simulink model "CSTR_sim_old"  (R2017a)
settings: Solver=ode8  StartTime=0.0  StopTime=t_end  FixedStep=Ts  RelTol=1e-3
values from neighbouring files (symbols this model uses):
  A = eval(A)    [linearisation.m]    (also in real_inverse.m = D * real( V' * diag( exp( j * angle( diag( V * D *  V.' ) ) )
  B = eval(B)    [linearisation.m]
  C = eval(C)    [linearisation.m]
  Ca = 1e-6    (= 1e-06)    [initialisation.m]    (also in linearisation.m = m.Ca; parameters.mat)
  Cb = 1e-6    (= 1e-06)    [initialisation.m]    (also in linearisation.m = m.Cb; parameters.mat)
  Fa0 = double(eval(S.Fa))    [linearisation.m]    (also in set_point.mat = 0.00260416666667)
  Fb0 = double(eval(S.Fb))    [linearisation.m]    (also in set_point.mat = 0.00572916666667)
  kv = 0.01    [initialisation.m]    (also in linearisation.m = m.kv; parameters.mat)
  kw = 1e-14    [initialisation.m]    (also in linearisation.m = m.kw; parameters.mat)
  tFa_down = 65000    [Simulation_Control_Off.m]
  tFa_up = 35000    [Simulation_Control_Off.m]
  tFb_down = 125000    [Simulation_Control_Off.m]
  tFb_up = 95000    [Simulation_Control_Off.m]
  V = 30    [initialisation.m]    (also in linearisation.m = m.V; parameters.mat)
  xa0 = 3.1250e-07    (= 3.125e-07)    [initialisation.m]    (also in linearisation.m = m.xa0; parameters.mat; set_point.mat)
  y = simdata.Data(:, 2)    [Simulation_Control_Off.m]    (also in initialisation.m = 7; linearisation.m = -log10(sqrt((xb - xa)^2/4 + kw) - (xb - xa)/2); parameters.mat = 7)
settings Model: Creator=Ivona  LastModifiedBy=Ivona

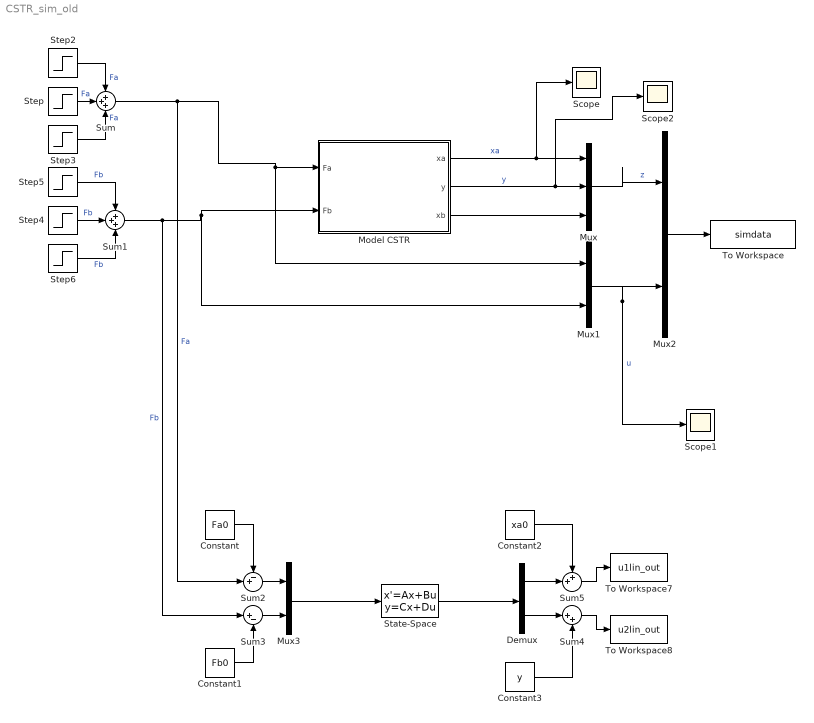
== system CSTR_sim_old ==
  Constant : Constant  Value=Fa0
  Constant1 : Constant  Value=Fb0
  Constant2 : Constant  Value=xa0
  Constant3 : Constant  Value=y
  Demux : Demux  Outputs=2
  Model CSTR : Subsystem
  Mux : Mux  Inputs=3
  Mux1 : Mux  Inputs=2
  Mux2 : Mux  Inputs=2
  Mux3 : Mux  Inputs=2
  Scope : Scope
  Scope1 : Scope
  Scope2 : Scope
  State-Space : StateSpace  A=A  B=B  C=C  D=[0 0;0 0]  X0=0
  Step : Step  Time=0  After=Fa0  SampleTime=0
  Step2 : Step  Time=tFa_up  After=0.1*Fa0  SampleTime=0
  Step3 : Step  Time=tFa_down  After=-0.1*Fa0  SampleTime=0
  Step4 : Step  Time=0  After=Fb0  SampleTime=0
  Step5 : Step  Time=tFb_up  After=0.1*Fb0  SampleTime=0
  Step6 : Step  Time=tFb_down  After=-0.1*Fb0  SampleTime=0
  Sum : Sum  Inputs=+++
  Sum1 : Sum  Inputs=+++
  Sum2 : Sum  Inputs=-+|
  Sum3 : Sum  Inputs=|+-
  Sum4 : Sum  Inputs=|++
  Sum5 : Sum  Inputs=++|
  To Workspace : ToWorkspace  VariableName=simdata  SaveFormat=Timeseries  SampleTime=-1
  To Workspace7 : ToWorkspace  VariableName=u1lin_out  SampleTime=-1
  To Workspace8 : ToWorkspace  VariableName=u2lin_out  SampleTime=-1
  wires:
  Model CSTR/1(xa) -> Mux/1, Scope/1  "xa"
  Model CSTR/2(y) -> Mux/2, Scope2/1  "y"
  Mux/1 -> Mux2/1  "z"
  Mux1/1 -> Scope1/1, Mux2/2  "u"
  Mux2/1 -> To Workspace/1
  Step/1 -> Sum/2  "Fa"
  Step2/1 -> Sum/1  "Fa"
  Step3/1 -> Sum/3  "Fa"
  Sum/1 -> Sum2/2, Mux1/1, Model CSTR/1(Fa)  "Fa"
  Step4/1 -> Sum1/2  "Fb"
  Step6/1 -> Sum1/3  "Fb"
  Step5/1 -> Sum1/1  "Fb"
  Sum1/1 -> Sum3/1, Mux1/2, Model CSTR/2(Fb)  "Fb"
  Model CSTR/3(xb) -> Mux/3
  Sum4/1 -> To Workspace8/1
  Constant2/1 -> Sum5/1
  Constant3/1 -> Sum4/2
  Constant1/1 -> Sum3/2
  Sum5/1 -> To Workspace7/1
  Constant/1 -> Sum2/1
  State-Space/1 -> Demux/1
  Demux/2 -> Sum4/1
  Sum2/1 -> Mux3/1
  Demux/1 -> Sum5/2
  Sum3/1 -> Mux3/2
  Mux3/1 -> State-Space/1

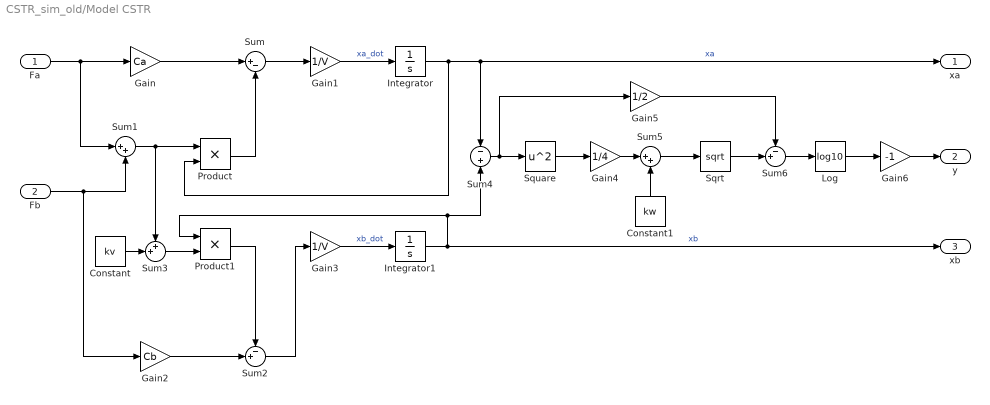
== system CSTR_sim_old/Model CSTR ==
  Fa : Inport
  Fb : Inport  Port=2
  Constant : Constant  Value=kv
  Constant1 : Constant  Value=kw
  Gain : Gain  Gain=Ca
  Gain1 : Gain  Gain=1/V
  Gain2 : Gain  Gain=Cb
  Gain3 : Gain  Gain=1/V
  Gain4 : Gain  Gain=1/4
  Gain5 : Gain  Gain=1/2
  Gain6 : Gain  Gain=-1
  Integrator : Integrator
  Integrator1 : Integrator
  Log : Math  Operator=log10  SaturateOnIntegerOverflow=on
  Product : Product
  Product1 : Product
  Sqrt : Sqrt  SaturateOnIntegerOverflow=on
  Square : Math  Operator=square  SaturateOnIntegerOverflow=on
  Sum : Sum  Inputs=|+-
  Sum1 : Sum  Inputs=|++
  Sum2 : Sum  Inputs=-+|
  Sum3 : Sum  Inputs=++|
  Sum4 : Sum  Inputs=-+
  Sum5 : Sum  Inputs=|++
  Sum6 : Sum  Inputs=-+|
  xa : Outport
  y : Outport  Port=2
  xb : Outport  Port=3
  wires:
  Integrator/1 -> Product/2, Sum4/1, xa/1  "xa"
  Fa/1 -> Sum1/1, Gain/1
  Gain/1 -> Sum/1
  Fb/1 -> Gain2/1, Sum1/2
  Sum1/1 -> Sum3/1, Product/1
  Product/1 -> Sum/2
  Sum/1 -> Gain1/1
  Gain1/1 -> Integrator/1  "xa_dot"
  Gain2/1 -> Sum2/2
  Constant/1 -> Sum3/2
  Product1/1 -> Sum2/1
  Sum2/1 -> Gain3/1
  Integrator1/1 -> xb/1, Sum4/2, Product1/1  "xb"
  Sum3/1 -> Product1/2
  Gain3/1 -> Integrator1/1  "xb_dot"
  Square/1 -> Gain4/1
  Gain4/1 -> Sum5/1
  Constant1/1 -> Sum5/2
  Sum5/1 -> Sqrt/1
  Sqrt/1 -> Sum6/2
  Gain5/1 -> Sum6/1
  Sum6/1 -> Log/1
  Log/1 -> Gain6/1
  Gain6/1 -> y/1
  Sum4/1 -> Gain5/1, Square/1
